simulink model "on_off_thruster"  (R2015b)
settings: Solver=VariableStepAuto  StartTime=0.0  StopTime=stop_time  RelTol=1e-6
values from neighbouring files (symbols this model uses):
  alpha_0 = alpha_0_deg*pi/180    (= 0.0174532925199)    [main_on_off_thruster.m]
  alpha_1 = alpha_1_deg*pi/180    (= 0.0523598775598)    [main_on_off_thruster.m]
  I_y = 0.5    [main_nonlinear_spacecraft_euler.m]    (also in main_nonlinear_spacecraft_quaternion.m; main_on_off_thruster.m; main_reaction_wheels_design_v02.m; main_reaction_wheels_design_v03.m)
  omega_y_0 = 0    [main_nonlinear_spacecraft_euler.m]    (also in main_nonlinear_spacecraft_quaternion.m; main_on_off_thruster.m; main_reaction_wheels_design_v03.m; main_reaction_wheels_design_v04.m)
  Q_0 = 0.1    [main_on_off_thruster.m]
  tau_y = k_d_y/k_p_y    (= 6.66666666667)    [main_on_off_thruster.m]
  theta_0 = 0    [main_nonlinear_spacecraft_euler.m]    (also in main_on_off_thruster.m = 2; main_reaction_wheels_design_v03.m = -0.3; main_reaction_wheels_design_v04.m = -0.10471975512)
settings Model: Creator=Krunal's PC  LastModifiedBy=Krunal's PC

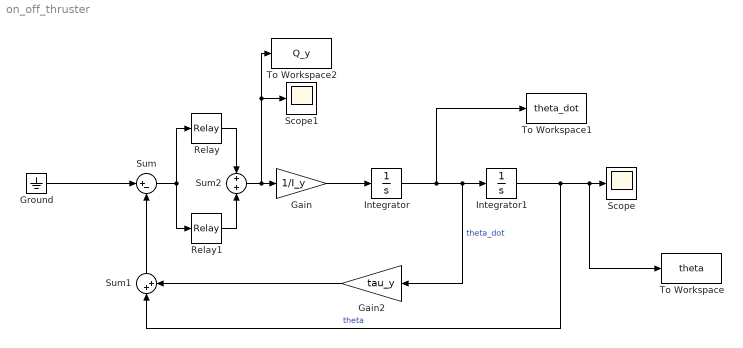
== system on_off_thruster ==
  Gain : Gain  Gain=1/I_y
  Gain2 : Gain  Gain=tau_y
  Ground : Ground
  Integrator : Integrator  InitialCondition=omega_y_0
  Integrator1 : Integrator  InitialCondition=theta_0
  Relay : Relay  OnSwitchValue=alpha_1  OffSwitchValue=alpha_0  OnOutputValue=Q_0
  Relay1 : Relay  OnSwitchValue=-alpha_0  OffSwitchValue=-alpha_1  OnOutputValue=0  OffOutputValue=-Q_0
  Scope : Scope
  Scope1 : Scope
  Sum : Sum  Inputs=|+-
  Sum1 : Sum  Inputs=|++
  Sum2 : Sum  Inputs=+|+
  To Workspace : ToWorkspace  VariableName=theta  SampleTime=-1
  To Workspace1 : ToWorkspace  VariableName=theta_dot  SampleTime=-1
  To Workspace2 : ToWorkspace  VariableName=Q_y  SampleTime=-1
  wires:
  Gain/1 -> Integrator/1
  Integrator/1 -> To Workspace1/1, Gain2/1, Integrator1/1  "theta_dot"
  Integrator1/1 -> Sum1/1, To Workspace/1, Scope/1  "theta"
  Gain2/1 -> Sum1/2
  Ground/1 -> Sum/1
  Sum1/1 -> Sum/2
  Sum/1 -> Relay1/1, Relay/1
  Relay1/1 -> Sum2/2
  Relay/1 -> Sum2/1
  Sum2/1 -> To Workspace2/1, Scope1/1, Gain/1
